simulink model "Mit_law"  (Simulink 7.3)
settings: Solver=ode5  StartTime=0.0  StopTime=200  FixedStep=0.01  RelTol=1e-3
StopFcn:
  | subplot(211);
  | plot(Data.time,Data.signals(1).values(:,1),'r',Data.time,Data.signals(1).values(:,2),'b')
  | subplot(212);
  | plot(Data.time,Data.signals(2).values(:,1),'b')
settings Model: Creator=Minh-Map-Vu  LastModifiedBy=nthuy
settings DataIOCC: SignalLoggingName=sigsOut
settings DebuggingCC: SaveWithParameterizedLinksMsg=none  SignalResolutionControl=TryResolveAllWithWarning  SolverPrmCheckMsg=none  MultiTaskDSMMsg=warning  MultiTaskCondExecSysMsg=none  StrictBusMsg=None
settings HardwareCC: TargetUnknown=on
settings RTWCC: IncludeERTFirstTime=on

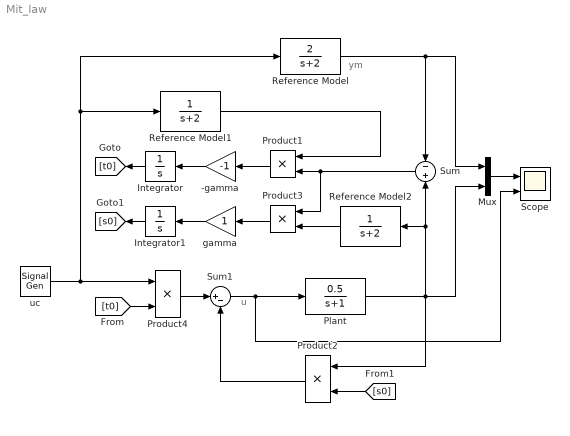
== system Mit_law ==
  note: ym
  note: u
  -gamma : Gain  Gain=-1  SaturateOnIntegerOverflow=on  OutDataTypeStr=Inherit: Same as input  ParamDataTypeStr=Inherit: Same as input
  Integrator : Integrator
  Integrator1 : Integrator
  Mux : Mux  Inputs=2
  Plant : TransferFcn  Numerator=0.5  Denominator=[1 1]
  Product{1..4} (4 alike) : Product  SaturateOnIntegerOverflow=on  OutDataTypeStr=Inherit: Same as first input
  Reference Model : TransferFcn  Numerator=[2]  Denominator=[1 2]
  Reference Model1 : TransferFcn  Numerator=1  Denominator=[1 2]
  Reference Model2 : TransferFcn  Numerator=1  Denominator=[1 2]
  Scope : Scope  NumInputPorts=2
      settings: TimeRange=100  YMin=-1.2~-5  YMax=1.2~5  SaveName=Data
  Sum : Sum  Inputs=-+  SaturateOnIntegerOverflow=on
  Sum1 : Sum  Inputs=|+-  SaturateOnIntegerOverflow=on
  gamma : Gain  SaturateOnIntegerOverflow=on  OutDataTypeStr=Inherit: Same as input  ParamDataTypeStr=Inherit: Same as input
  uc : SignalGenerator  WaveForm=square  Frequency=1/20
  wires:
  uc/1 -> Reference Model/1, Reference Model1/1, Product4/1
  Reference Model/1 -> Sum/1, Mux/1
  Sum1/1 -> Plant/1, Scope/2
  -gamma/1 -> Integrator/1
  Product4/1 -> Sum1/1
  Plant/1 -> Mux/2, Product2/1, Sum/2, Reference Model2/1
  Product1/1 -> -gamma/1
  Sum/1 -> Product1/2, Product3/1
  Mux/1 -> Scope/1
  Integrator/1 -> [t0]
  [t0] -> Product4/2
  [s0] -> Product2/2
  Product2/1 -> Sum1/2
  Reference Model1/1 -> Product1/1
  Reference Model2/1 -> Product3/2
  Product3/1 -> gamma/1
  Integrator1/1 -> [s0]
  gamma/1 -> Integrator1/1
